simulink model "ImportTemperature"  (R2022b)
settings: Solver=VariableStepAuto  StartTime=0.0  StopTime=744  RelTol=1e-3
settings Model: Creator=jim  LastModifiedBy=jim

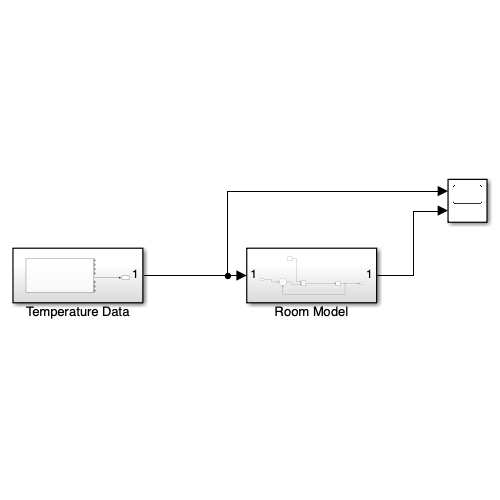
[thumbnail: Simulink's stored preview of the top-level diagram]
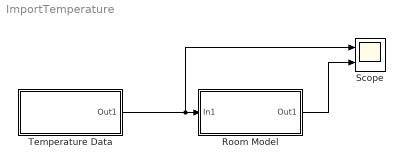
== system ImportTemperature ==
  Room Model : Subsystem
  Scope : Scope  NumInputPorts=2
  Temperature Data : Subsystem
  wires:
  Temperature Data/1(Out1) -> Room Model/1(In1), Scope/1
  Room Model/1(Out1) -> Scope/2

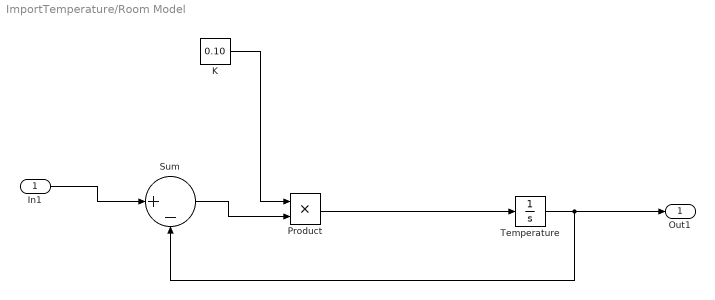
== system ImportTemperature/Room Model ==
  In1 : Inport
  K : Constant  Value=0.10
  Product : Product
  Sum : Sum  Inputs=|+-
  Temperature : Integrator  InitialCondition=20
  Out1 : Outport
  wires:
  In1/1 -> Sum/1
  Temperature/1 -> Sum/2, Out1/1
  Product/1 -> Temperature/1
  K/1 -> Product/1
  Sum/1 -> Product/2

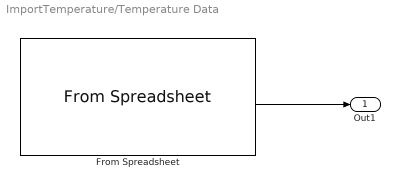
== system ImportTemperature/Temperature Data ==
  From Spreadsheet : FromSpreadsheet  FileName=/Users/jim/Dropbox/GitHub Clones/CT549/code/04_Lecture/01 Temperature/A17_MACE HEAD_M10.xlsx  SheetName=A17_MACE HEAD_M10
  Out1 : Outport
  wires:
  From Spreadsheet/5 -> Out1/1
